simulink model "FG_RealTime_original"  (R2017b)
settings: Solver=FixedStepDiscrete  StartTime=0.0  StopTime=inf  FixedStep=UserParams.SampleTime  RelTol=1e-3  EnableMultiTasking=on
InitFcn:
  | isSim = 0;
  | PreFunctions.CustomInitFcn;
undefined symbols (not defined in the file or in its folder): BusModule, getLinuxDataStruct, getSlrtDataStruct
libraries: slrtlib x3, FG_Controller_Library x2, xpcrtudplib x2, CassieLibrary x1
settings Model: xpc_rtwmakecfg_data=_xpcethercatlib_  TunableVars=c_CP_StanceAbdu,c_CP_StanceKnee,c_CP_SwingAbdu,c_CP_SwingKnee,c_Gamma_knee,c_Gamma_st_abu,c_Gamma_st_hip,c_Gamma_st_knee,c_Gamma_sw_abu,c_Gamma_sw_hip,c_Gamma_sw_knee,c_Kd_abduction,c_Kd_abduction_stand,c_Kd_knee,c_Kd_knee_stand,c_Kd_lateral_stand,c_Kd_pitch,c_Kd_roll,c_Kd_rotation,c_Kd_rotation_stand,c_Kd_thigh,c_Kd_thigh_stand,c_Kd_toe,c_Kd_toe_stand,c_Kd_yaw,c_Kfl_d,c_Kfl_p,c_Kfs_d,c_Kfs_p,c_Kp_abduction,c_Kp_abduction_stand,c_Kp_knee,c_Kp_knee_stand,c_Kp_lateral_stand,c_Kp_pitch,c_Kp_roll,c_Kp_rotation,c_Kp_rotation_stand,c_Kp_thigh,c_Kp_thigh_stand,c_Kp_toe,c_Kp_toe_stand,c_Kp_yaw,c_abduction_inward_gain,c_com_bp,c_fil_para_2,c_fil_para_3,c_fil_para_4,c_fil_para_5,c_fil_para_x,c_fil_para_y,c_fil_vel_offset,c_final_st_abduction,c_final_sw_abduction,c_force_step_end_s,c_init_lateral_velocity,c_joint_filter_choice,c_lateral_offset_exp,c_lateral_velocity_weight,c_pre_final_sw_abduction,c_sagittal_offset_exp,c_sagittal_speed,c_shift_distance,c_shift_time,c_stance_thre_lb,c_stance_thre_ub,c_stand_offset_exp,c_standing_switch_time,c_toe_tilt_angle,c_turning_offset_exp,c_u_abduction_cp,c_u_abduction_swing_cp,c_u_knee_cp,c_u_thigh_cp  TunableVarsStorageClass=Auto,Auto,Auto,Auto,Auto,Auto,Auto,Auto,Auto,Auto,Auto,Auto,Auto,Auto,Auto,Auto,Auto,Auto,Auto,Auto,Auto,Auto,Auto,Auto,Auto,Auto,Auto,Auto,Auto,Auto,Auto,Auto,Auto,Auto,Auto,Auto,Auto,Auto,Auto,Auto,Auto,Auto,Auto,Auto,Auto,Auto,Auto,Auto,Auto,Auto,Auto,Auto,Auto,Auto,Auto,Auto,Auto,Auto,Auto,Auto,Auto,Auto,Auto,Auto,Auto,Auto,Auto,Auto,Auto,Auto,Auto,Auto,Auto,Auto  TunableVarsTypeQualifier=,,,,,,,,,,,,,,,,,,,,,,,,,,,,,,,,,,,,,,,,,,,,,,,,,,,,,,,,,,,,,,,,,,,,,,,,,  Creator=robot  LastModifiedBy=RoahmLab
settings SolverCC: ConcurrentTasks=on
settings DataIOCC: SaveFormat=Array  SaveOutput=off  SignalLogging=off  DSMLogging=off  VisualizeSimOutput=off  SaveTime=off
settings OptimizationCC: LifeSpan=inf  SimCompilerOptimization=on  AccelVerboseBuild=on
settings DebuggingCC: AllowSymbolicDim=off  SFUnexpectedBacktrackingDiag=warning  SFNoUnconditionalDefaultTransitionDiag=warning  SFExecutionAtInitializationDiag=none
settings HardwareCC: ProdBitPerPointer=32  ProdBitPerSizeT=32  ProdBitPerPtrDiffT=32  ProdLargestAtomicFloat=None  ProdWordSize=32  ProdLongLongMode=on  ProdHWDeviceType=Generic->32-bit x86 compatible
settings ModelReferenceCC: ParallelModelReferenceMATLABWorkerInit=Copy Base Workspace  ModelReferenceNumInstancesAllowed=Zero  PropagateSignalLabelsOutOfModel=off
settings SFSimCC: SimUserIncludeDirs=D:\Graduate\robots\Cassie\GitHub\Cassie_Controller_V3_Yukai\Controllers\Flatground\utils\funcs\kin  SFSimEcho=off
settings SFSimCC: SimUserSources=|
  | ComPosition_src.c
  | ComVelocity_src.c
  | J_LeftToeBottomBack_src.c
  | J_LeftToeBottomFront_src.c
  | J_LeftToeBottom_src.c
  | J_LeftToeJoint_src.c
  | J_RightToeBottomBack_src.c
  | J_RightToeBottomFront_src.c
  | J_RightToeBottom_src.c
  | J_RightToeJoint_src.c
  | LeftToeBottomBack_src.c
  | LeftToeBottomFront_src.c
  | LeftToeBottom_src.c
  | LeftToeJoint_src.c
  | RightToeBottomBack_src.c
  | RightToeBottomFront_src.c
  | RightToeBottom_src.c
  | RightToeJoint_src.c
settings RTWCC: SystemTargetFile=slrt.tlc  TLCOptions=-axPCMaxOverloads=1000000000 -axPCMaxOverloadLen=1000000000  TemplateMakefile=slrt_default_tmf  Description=Simulink Real-Time  RTWUseSimCustomCode=on  CustomInclude=D:\Graduate\robots\Cassie\GitHub\Cassie_Controller_V3_Yukai\Controllers\Flatground\utils\funcs\kin  CodeExecutionProfiling=on  CodeProfilingSaveOptions=AllData  CodeProfilingInstrumentation=on  RTWCompilerOptimization=on
settings RTWCC: CustomSource=|
  | ComPosition_src.c
  | ComVelocity_src.c
  | J_LeftToeBottomBack_src.c
  | J_LeftToeBottomFront_src.c
  | J_LeftToeBottom_src.c
  | J_LeftToeJoint_src.c
  | J_RightToeBottomBack_src.c
  | J_RightToeBottomFront_src.c
  | J_RightToeBottom_src.c
  | J_RightToeJoint_src.c
  | LeftToeBottomBack_src.c
  | LeftToeBottomFront_src.c
  | LeftToeBottom_src.c
  | LeftToeJoint_src.c
  | RightToeBottomBack_src.c
  | RightToeBottomFront_src.c
  | RightToeBottom_src.c
  | RightToeJoint_src.c
settings CodeAppCC: GenerateComments=off  MaxIdLength=128  SimulinkBlockComments=off
settings ConfigComp: CovMetricSettings=dw  CovHtmlReporting=on  CovSaveCumulativeToWorkspaceVar=on  CovSaveSingleToWorkspaceVar=on  CovExternalEMLEnable=off

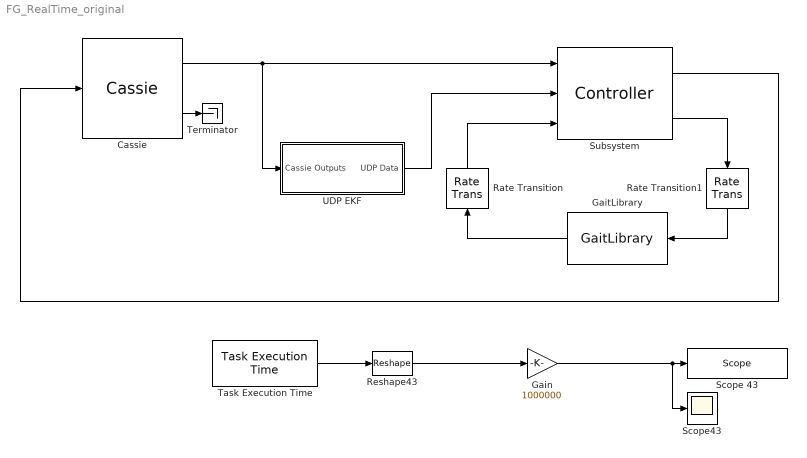
== system FG_RealTime_original ==
  Cassie : CassieLibrary/RealTime/Cassie  SystemSampleTime=-1
  Gain : Gain  Gain=1000000
  GaitLibrary : FG_Controller_Library/GaitLibrary
  Rate Transition : RateTransition  Deterministic=off  OutPortSampleTime=UserParams.SampleTime
  Rate Transition1 : RateTransition  Deterministic=off  OutPortSampleTime=0.1
  Reshape43 : Reshape
  Scope 43 : slrtlib/Displays and Logging/Scope   scopeno=1  scopetype=Host  autostart=on  viewmode=Graphical redraw  formatstr='%15.6f'  grid=on  ylimits=[0,0]  nosamples=2500  noprepostsamples=0  interleave=1  triggermode=FreeRun  triggersignal=1  trigsignalfromport=off  triggerlevel=0.0  triggerslope=Either  triggerscope=1  triggersample=0  filename=data.dat  mode=Lazy  writesize=512  autorestart=off  dynamicfilemode=off  maxwritefilesize=512*1024^2
  Scope43 : Scope
  Subsystem : FG_Controller_Library/Controller
  "Task Execution Time " : slrtlib/Target Management/Execution Parameters/Task Execution Time   ts=0.0005
      settings: SourceProductName=Simulink Real-Time  SourceProductBaseCode=XP
  Terminator : Terminator
  UDP EKF : Subsystem
  wires:
  Subsystem/1 -> Cassie/1
  Cassie/1 -> UDP EKF/1(Cassie Outputs), Subsystem/1
  UDP EKF/1(UDP Data) -> Subsystem/2
  Cassie/2 -> Terminator/1
  Subsystem/2 -> Rate Transition1/1
  GaitLibrary/1 -> Rate Transition/1
  Rate Transition/1 -> Subsystem/3
  Rate Transition1/1 -> GaitLibrary/1
  Reshape43/1 -> Gain/1
  "Task Execution Time "/1 -> Reshape43/1
  Gain/1 -> Scope43/1, Scope 43/1

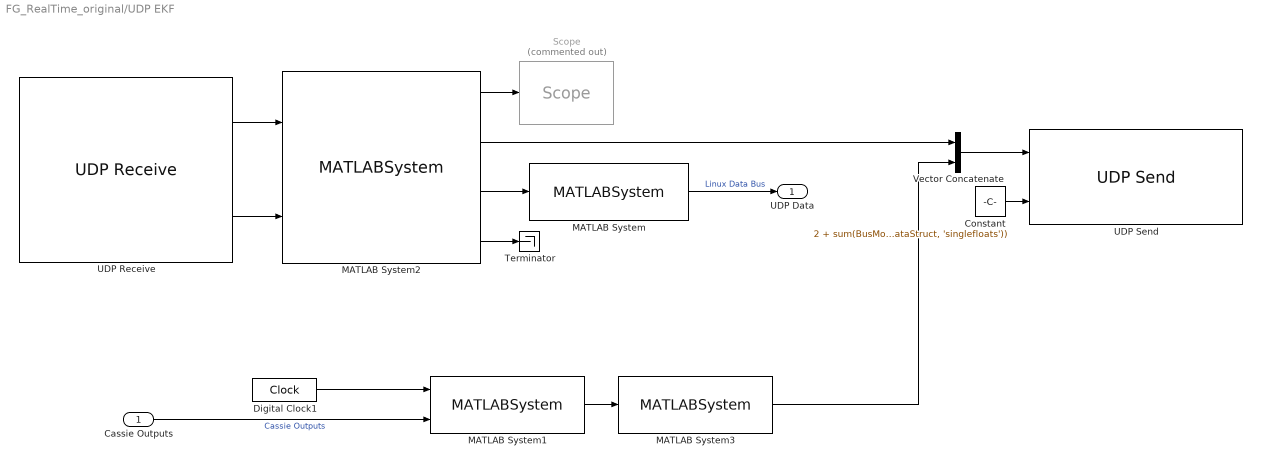
== system FG_RealTime_original/UDP EKF ==
  Cassie Outputs : Inport
  Constant : Constant  Value=2 + sum(BusModule.getPackingInfo(getSlrtDataStruct, 'singlefloats'))
  Digital Clock1 : DigitalClock  SampleTime=-1
  MATLAB System : MATLABSystem  System=BytesToCassieLinuxDataBus  SimulateUsing=Code generation
      mask Type: BytesToCassieLinuxDataBus
      mask Display: disp('BytesToCassieLinuxDataBus');
  MATLAB System1 : MATLABSystem  System=ConstructSlrtDataBus  SimulateUsing=Code generation
      mask Type: ConstructSlrtDataBus
      mask Display:
      | disp('ConstructSlrtDataBus');
      | port_label('input',1,'t');
      | port_label('input',2,'outputs');
      | port_label('output',1,'data');
  MATLAB System2 : MATLABSystem  System=ProcessUdpPacket  heartbeatInterval=0.01  HeaderLength=2  CassieLinuxDataLength=sum(BusModule.getPackingInfo(getLinuxDataStruct, 'singlefloats'))  SimulateUsing=Code generation
      mask Type: ProcessUdpPacket
      mask Display:
      | disp('ProcessUdpPacket');
      | port_label('input',1,'UDP Data');
      | port_label('input',2,'Length');
      | port_label('output',1,'Log');
      | port_label('output',2,'Header');
      | port_label('output',3,'LinuxData');
      | port_label('output',4,'timeout');
  MATLAB System3 : MATLABSystem  System=CassieSlrtDataBusToBytes  SimulateUsing=Code generation
      mask Type: CassieSlrtDataBusToBytes
      mask Display: disp('CassieSlrtDataBusToBytes');
  "Scope " : slrtlib/Displays and Logging/Scope   Commented=on  scopeno=1  scopetype=File  autostart=on  viewmode=Graphical redraw  formatstr='%15.6f'  grid=on  ylimits=[0,0]  nosamples=250  noprepostsamples=0  interleave=1  triggermode=FreeRun  triggersignal=1  trigsignalfromport=off  triggerlevel=0.0  triggerslope=Either  triggerscope=1  triggersample=0  filename=udp.dat  mode=Commit  writesize=4096  autorestart=on  dynamicfilemode=off  maxwritefilesize=2048*1024^2 - 4096
  Terminator : Terminator
  UDP Receive : xpcrtudplib/UDP Receive  ipAddressVal=Use host-target connection  localPort=25000  rcvWidth=2 + sum(BusModule.getPackingInfo(getLinuxDataStruct, 'singlefloats'))  rcvFmAny=off  fmAddress=10.10.10.5  maxUDPQueue=8  sampleTime=-1
      settings: SourceProductName=Simulink Real-Time
  UDP Send : xpcrtudplib/UDP Send  ipAddressVal=Use host-target connection  localPort=-1  toAddress=10.10.10.5  toPort=26000  sampleTime=0.0005
      settings: SourceProductName=Simulink Real-Time  SourceProductBaseCode=XP
  Vector Concatenate : Concatenate
  UDP Data : Outport
  wires:
  MATLAB System1/1 -> MATLAB System3/1
  MATLAB System2/3 -> MATLAB System/1
  MATLAB System2/1 -> "Scope "/1
  Digital Clock1/1 -> MATLAB System1/1
  UDP Receive/2 -> MATLAB System2/2
  MATLAB System3/1 -> Vector Concatenate/2
  UDP Receive/1 -> MATLAB System2/1
  Constant/1 -> UDP Send/2
  Vector Concatenate/1 -> UDP Send/1
  MATLAB System2/2 -> Vector Concatenate/1
  MATLAB System/1 -> UDP Data/1  "Linux Data Bus"
  MATLAB System2/4 -> Terminator/1
  Cassie Outputs/1 -> MATLAB System1/2  "Cassie Outputs"
